simulink model "disenyo_filtro"  (R2021a)
settings: Solver=FixedStepAuto  StartTime=0.0  StopTime=Inf  FixedStep=0.01  RelTol=1e-3  EnableMultiTasking=on
libraries: simulink x2, arduinolib x2, dspstat3 x1
settings Model: SILPILModeSetting=veronly  ExtModeTrigDuration=2  Creator=Simón  LastModifiedBy=Simón
settings OptimizationCC: EnhancedBackFolding=on  PassReuseOutputArgsAs=Individual arguments  ZeroExternalMemoryAtStartup=off  ZeroInternalMemoryAtStartup=off  MaxStackSize=64  OptimizeBlockOrder=speed  DifferentSizesBufferReuse=on  OptimizationCustomize=off  EfficientTunableParamExpr=on
settings DebuggingCC: ParameterTunabilityLossMsg=error
settings HardwareCC: ProdBitPerInt=16  ProdBitPerPointer=16  ProdBitPerSizeT=16  ProdBitPerPtrDiffT=16  ProdLargestAtomicFloat=None  ProdWordSize=8  ProdHWDeviceType=Atmel->AVR  UseEmbeddedCoderFeatures=off  UseSimulinkCoderFeatures=off
settings SFSimCC: MATLABDynamicMemAlloc=off
settings RTWCC: SystemTargetFile=ert.tlc  HardwareBoard=Arduino Uno  TemplateMakefile=ert_default_tmf  Toolchain=Arduino AVR  BuildConfiguration=Faster Runs
settings CodeAppCC: ForceParamTrailComments=on  IgnoreCustomStorageClasses=off  OperatorAnnotations=on  SimulinkDataObjDesc=on  SFDataObjDesc=on  InsertBlockDesc=on
settings ERTTargetCC: SupportContinuousTime=on  SupportNonInlinedSFcns=on  SupportVariableSizeSignals=on  ExtModeStaticAllocSize=250

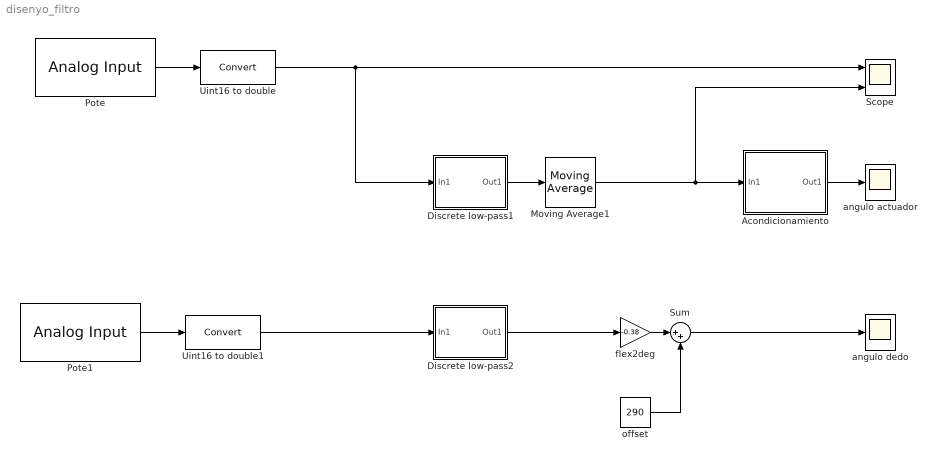
== system disenyo_filtro ==
  Acondicionamiento : Subsystem
  Discrete low-pass1 : Subsystem
  Discrete low-pass2 : Subsystem
  Moving Average1 : dspstat3/Moving Average  Method=Sliding window  ForgettingFactorPort=off  SpecifyWindowLength=on  WindowLength=5  ForgettingFactor=0.9  SimulateUsing=Code generation
  Pote : arduinolib/Analog Input  pinNumber=0  ReadResultsOnly=off  ConversionTriggerSource=Software  ExternalTriggerType=uint32( 0 )  OutputDataType=uint16  EnableConversionCompleteNotify=off  EnableOuputStatus=off  SampleTime=-1  blockPlatform=arduino
  Pote1 : arduinolib/Analog Input  pinNumber=1  ReadResultsOnly=off  ConversionTriggerSource=Software  ExternalTriggerType=uint32( 0 )  OutputDataType=uint16  EnableConversionCompleteNotify=off  EnableOuputStatus=off  SampleTime=-1  blockPlatform=arduino
  Scope : Scope  NumInputPorts=2
  Sum : Sum  Inputs=|++
  Uint16 to double : DataTypeConversion
  Uint16 to double1 : DataTypeConversion
  angulo actuador : Scope
  angulo dedo : Scope
  flex2deg : Gain  Gain=-0.38
  offset : Constant  Value=290
  wires:
  Pote/1 -> Uint16 to double/1
  Uint16 to double/1 -> Discrete low-pass1/1(In1), Scope/1
  Discrete low-pass1/1(Out1) -> Moving Average1/1
  Moving Average1/1 -> Acondicionamiento/1(In1), Scope/2
  flex2deg/1 -> Sum/1
  offset/1 -> Sum/2
  Sum/1 -> angulo dedo/1
  Pote1/1 -> Uint16 to double1/1
  Uint16 to double1/1 -> Discrete low-pass2/1(In1)
  Discrete low-pass2/1(Out1) -> flex2deg/1
  Acondicionamiento/1(Out1) -> angulo actuador/1

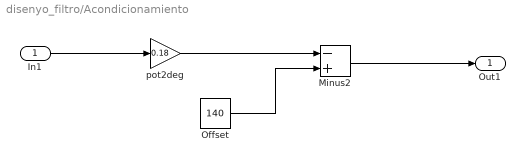
== system disenyo_filtro/Acondicionamiento ==
  In1 : Inport
  Minus2 : Sum  Inputs=-+
  Offset : Constant  Value=140
  pot2deg : Gain  Gain=0.18
  Out1 : Outport
  wires:
  Offset/1 -> Minus2/2
  In1/1 -> pot2deg/1
  pot2deg/1 -> Minus2/1
  Minus2/1 -> Out1/1

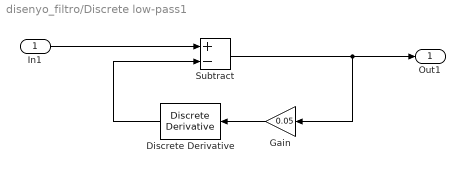
== system disenyo_filtro/Discrete low-pass1 ==
  In1 : Inport
  Discrete Derivative : simulink/Discrete/Discrete Derivative  gainval=1.0  ICPrevScaledInput=0.0  OutMin=[]  OutMax=[]  OutDataType=fixdt(1, 16)  OutScaling=2^-10  DoSatur=off
  Gain : Gain  Gain=0.05
  Subtract : Sum  Inputs=+-
  Out1 : Outport
  wires:
  Discrete Derivative/1 -> Subtract/2
  Subtract/1 -> Out1/1, Gain/1
  Gain/1 -> Discrete Derivative/1
  In1/1 -> Subtract/1

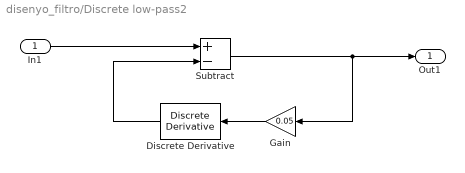
== system disenyo_filtro/Discrete low-pass2 ==
  In1 : Inport
  Discrete Derivative : simulink/Discrete/Discrete Derivative  gainval=1.0  ICPrevScaledInput=0.0  OutMin=[]  OutMax=[]  OutDataType=fixdt(1, 16)  OutScaling=2^-10  DoSatur=off
  Gain : Gain  Gain=0.05
  Subtract : Sum  Inputs=+-
  Out1 : Outport
  wires:
  In1/1 -> Subtract/1
  Gain/1 -> Discrete Derivative/1
  Subtract/1 -> Gain/1, Out1/1
  Discrete Derivative/1 -> Subtract/2
